simulink model "TDMA_sim_TxRx2020"  (R2016a)
settings: Solver=ode45  StartTime=0.0  StopTime=20  MaxStep=.01  MinStep=.001  RelTol=1e-3
libraries: dsparch4 x2
settings Model: Creator=user  LastModifiedBy=Simona
settings DataIOCC: LimitDataPoints=on  SaveFormat=Array  SignalLoggingSaveFormat=ModelDataLogs
settings OptimizationCC: ExpressionDepthLimit=2147483647  InitFltsAndDblsToZero=on
settings DebuggingCC: SaveWithParameterizedLinksMsg=none  UnderspecifiedInitializationDetection=Classic  MergeDetectMultiDrivingBlocksExec=none  SolverPrmCheckMsg=warning  FcnCallInpInsideContextMsg=UseLocalSettings  StateNameClashWarn=warning
settings HardwareCC: ProdBitPerPointer=32  ProdLargestAtomicFloat=None  ProdIntDivRoundTo=Undefined  ProdEndianess=Unspecified  ProdWordSize=32  ProdHWDeviceType=32-bit Generic
settings ModelReferenceCC: PropagateSignalLabelsOutOfModel=off
settings GRTTargetCC: CombineOutputUpdateFcns=off  GRTInterface=on
settings ConfigComp: CovModelRefEnable=Off

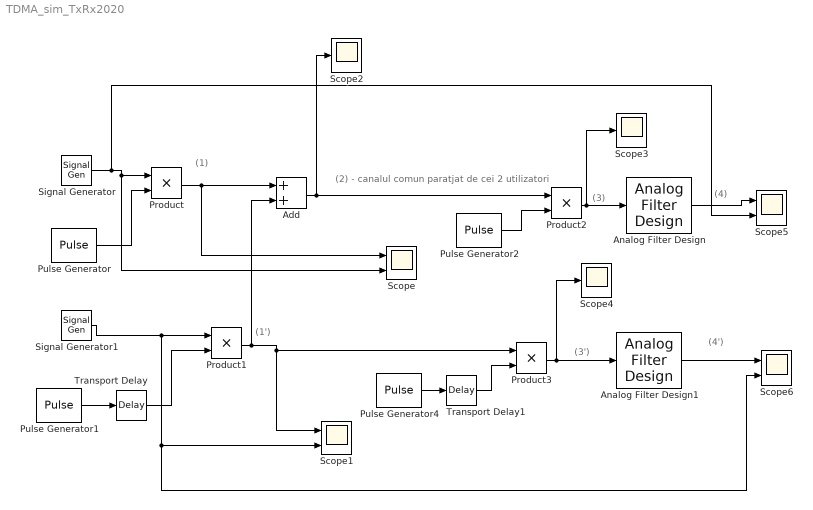
== system TDMA_sim_TxRx2020 ==
  note: (1)
  note: (1')
  note: (2) - canalul comun paratjat de cei 2 utilizatori
  note: (3)
  note: (3')
  note: (4)
  note: (4')
  Add : Sum
  Analog Filter Design : dsparch4/Analog Filter Design  method=Butterworth  filttype=Lowpass  N=10  Wlo=2*2*pi  Whi=80  Rp=2  Rs=40
  Analog Filter Design1 : dsparch4/Analog Filter Design  method=Butterworth  filttype=Lowpass  N=10  Wlo=4*2*pi  Whi=80  Rp=2  Rs=40
  Product{,1..3} (4 alike) : Product  RndMeth=Zero
  Pulse Generator{,1..2,4} (4 alike) : DiscretePulseGenerator  PulseType=Time based  Period=.4  PulseWidth=50
  Scope{,1,5..6} (4 alike) : Scope  NumInputPorts=2
  Scope2 : Scope
  Scope3 : Scope
  Scope4 : Scope
  Signal Generator : SignalGenerator  WaveForm=square  Frequency=.25
  Signal Generator1 : SignalGenerator  Frequency=.25
  Transport Delay : TransportDelay  DelayTime=.2
  Transport Delay1 : TransportDelay  DelayTime=.22
  wires:
  Pulse Generator1/1 -> Transport Delay/1
  Signal Generator/1 -> Product/1, Scope/2, Scope5/2
  Pulse Generator/1 -> Product/2
  Product/1 -> Scope/1, Add/1
  Signal Generator1/1 -> Product1/1, Scope1/2, Scope6/2
  Transport Delay/1 -> Product1/2
  Product1/1 -> Add/2, Scope1/1, Product3/1
  Add/1 -> Scope2/1, Product2/1
  Pulse Generator2/1 -> Product2/2
  Product2/1 -> Scope3/1, Analog Filter Design/1
  Product3/1 -> Scope4/1, Analog Filter Design1/1
  Pulse Generator4/1 -> Transport Delay1/1
  Transport Delay1/1 -> Product3/2
  Analog Filter Design/1 -> Scope5/1
  Analog Filter Design1/1 -> Scope6/1
